simulink model "pid_control"  (R2022a)
settings: Solver=ode4  StartTime=0.0  StopTime=15  FixedStep=0.002  RelTol=1e-3
InitFcn:
  | num=1;
  | den=[1 1 1];  % 2nd order plant model
values from neighbouring files (symbols this model uses):
  Kd = K(i)    [PD_control_script.m]    (also in PD_only.m = 5)
  Ki = K(i)    [PI_only.m]    (also in Pi_control_script.m; i_control_script.m)
  Kp = 1    [PD_control_script.m]    (also in PD_only.m; PI_only.m; Pi_control_script.m; p_control_script.m = K(i))
  N = 100    [PD_control_script.m]    (also in PD_only.m = Ni(i))
libraries: slpidlib x1
settings Model: Creator=김응태  LastModifiedBy=ADMIN

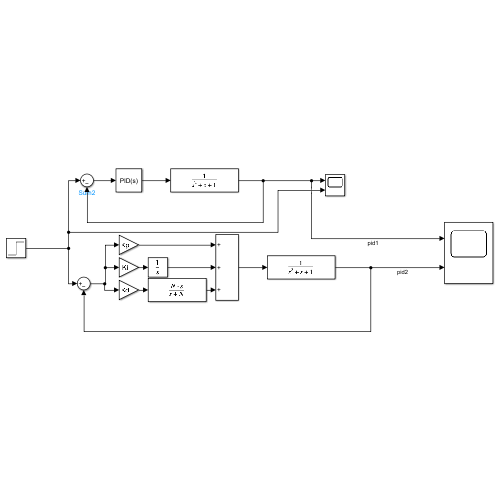
[thumbnail: Simulink's stored preview of the top-level diagram]
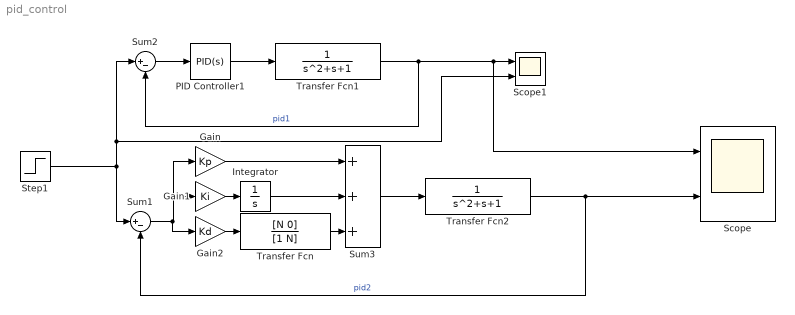
== system pid_control ==
  Gain : Gain  Gain=Kp
  Gain1 : Gain  Gain=Ki
  Gain2 : Gain  Gain=Kd
  Integrator : Integrator
  PID Controller1 : slpidlib/PID Controller  Controller=PID  Form=Parallel  TimeDomain=Continuous-time  UseExternalTs=off  SampleTime=-1  IntegratorMethod=Forward Euler  FilterMethod=Forward Euler  ControllerParametersSource=internal  P=10.859494894698  I=5.7133780114071  UseKiTs=off  D=4.97921968501972  N=30.1310064984328  UseFilter=on  TunerSelectOption=Transfer Function Based (PID Tuner App)  InitialConditionSource=internal  InitialConditionForIntegrator=0  InitialConditionForFilter=0  DifferentiatorICPrevScaledInput=0  ExternalReset=none  TrackingMode=off  Kt=1  LimitOutput=off  SatLimitsSource=internal  UpperSaturationLimit=inf  LowerSaturationLimit=-inf  LinearizeAsGain=on  AntiWindupMode=none  Kb=1  POutMin=[]  POutMax=[]  IOutMin=[]  IOutMax=[]  DOutMin=[]  DOutMax=[]  NOutMin=[]  NOutMax=[]  SumOutMin=[]  SumOutMax=[]  SaturationOutMin=[]  SaturationOutMax=[]  PParamMin=[]  PParamMax=[]  IParamMin=[]  IParamMax=[]  DParamMin=[]  DParamMax=[]  NParamMin=[]  NParamMax=[]  KbParamMin=[]  KbParamMax=[]  KtParamMin=[]  KtParamMax=[]  KbOutMin=[]  KbOutMax=[]  KtOutMin=[]  KtOutMax=[]  IntegratorOutMin=[]  IntegratorOutMax=[]  FilterOutMin=[]  FilterOutMax=[]  SumI1OutMin=[]  SumI1OutMax=[]  SumI2OutMin=[]  SumI2OutMax=[]  SumI3OutMin=[]  SumI3OutMax=[]  SumI4OutMin=[]  SumI4OutMax=[]  SumDOutMin=[]  SumDOutMax=[]  DifferentiatorOutMin=[]  DifferentiatorOutMax=[]  FilterDiffOutCoefMin=[]  FilterDiffOutCoefMax=[]  ReciprocalOutMin=[]  ReciprocalOutMax=[]  SumDenOutMin=[]  SumDenOutMax=[]  SumNumOutMin=[]  SumNumOutMax=[]  DivideOutMin=[]  DivideOutMax=[]  UdiffTsProdOutMin=[]  UdiffTsProdOutMax=[]  NTsProdOutMin=[]  NTsProdOutMax=[]  UintegralTsProdOutMin=[]  UintegralTsProdOutMax=[]  UngainTsProdOutMin=[]  UngainTsProdOutMax=[]  IntegratorContinuousStateAttributes=''  IntegratorStateMustResolveToSignalObject=off  IntegratorRTWStateStorageClass=Auto  FilterContinuousStateAttributes=''  FilterStateMustResolveToSignalObject=off  FilterRTWStateStorageClass=Auto  ParallelPVariant=InternalParameters  IdealPVariant=Disabled  IVariant=InternalParameters  DVariant=InternalParameters  IntegratorVariant=Continuous  SatVariant=Disabled  AWVariant=Passthrough  PCopyVariant=Disabled  TRVariant=Disabled  FdbkBlocksVariant=Forward  IdealPFdbkVariant=Disabled  SatFdbkVariant=Disabled  DerivativeFilterVariant=ContFilter  NVariant=InternalParameters  NCopyVariant=Disabled  FilterICVariant=InternalICsFilter  IntegratorICVariant=InternalICs  ExternalResetVariant=Disabled  TRSumVariant=Passthrough  SumFdbkVariant=Disabled  SumVariant=Sum_PID  TsampFilterVariant=InternalTs  TsampNgainVariant=Passthrough  TsampIntegralVariant=Passthrough  ExternalSaturationOutDataTypeStr=Inherit: Same as second input  aMode=0
  Scope : Scope  NumInputPorts=2
  Scope1 : Scope  NumInputPorts=2
  Step1 : Step  SampleTime=0
  Sum1 : Sum  Inputs=|+-
  Sum2 : Sum  Inputs=|+-
  Sum3 : Sum  Inputs=+++
  Transfer Fcn : TransferFcn  Numerator=[N 0]  Denominator=[1 N]
  Transfer Fcn1 : TransferFcn  Numerator=1  Denominator=[1 1 1]
  Transfer Fcn2 : TransferFcn  Numerator=1  Denominator=[1 1 1]
  wires:
  Sum2/1 -> PID Controller1/1
  PID Controller1/1 -> Transfer Fcn1/1
  Transfer Fcn1/1 -> Sum2/2, Scope/1, Scope1/1  "pid1"
  Step1/1 -> Sum1/1, Sum2/1, Scope1/2
  Transfer Fcn2/1 -> Sum1/2, Scope/2  "pid2"
  Sum3/1 -> Transfer Fcn2/1
  Sum1/1 -> Gain2/1, Gain1/1, Gain/1
  Gain/1 -> Sum3/1
  Gain1/1 -> Integrator/1
  Integrator/1 -> Sum3/2
  Gain2/1 -> Transfer Fcn/1
  Transfer Fcn/1 -> Sum3/3
